simulink model "LV_grid"  (R2021b)
settings: Solver=VariableStepAuto  StartTime=0  StopTime=5.0005  FixedStep=5e-4  RelTol=1e-3
model workspace (MAT data in the model file):
  P2_1 = 3450
  idx = 1
  time_counter = 1
libraries: spsGroundLib x97, spsStairGeneratorLib x96, spsPiSectionLineLib x90, spsThreePhasePISectionLineLib x90, spsVariableInductorLib x48, spsVariableResistorLib x48, spsRMSLib x36, spsThreePhaseVIMeasurementLib x34, spsACVoltageSourceLib x5, spsLinearTransformerLib x5, spsPower3phInstantaneousLib x1, spsThreePhaseMutualInductanceZ1Z0Lib x1
(part 3 of 6)

== system LV_grid/L25 ==
  note: 2.5m
  note: 2.5m
  note: 2.5m
  note: 2.5m
  Ground : spsGroundLib/Ground  LConnTagsString=a
  Ground1 : spsGroundLib/Ground  LConnTagsString=a
  Ground2 : spsGroundLib/Ground  LConnTagsString=a
  L1 : Subsystem
  L2 : Subsystem
  L3 : Subsystem
  L4 : Subsystem
  A : PMIOPort  Side=Left
  B : PMIOPort  Port=2  Side=Left
  C : PMIOPort  Port=3  Side=Left
  N : PMIOPort  Port=4  Side=Left
  a : PMIOPort  Port=5  Side=Right
  b : PMIOPort  Port=6  Side=Right
  c : PMIOPort  Port=7  Side=Right
  n : PMIOPort  Port=8  Side=Right
  connections:
  L1/LConn3 -- C/RConn1
  L3/LConn4 -- Ground1/LConn1 -- L2/RConn4
  L1/LConn4 -- N/RConn1
  L1/LConn2 -- B/RConn1
  L1/LConn1 -- A/RConn1
  L2/LConn4 -- Ground/LConn1 -- L1/RConn4
  L4/LConn4 -- Ground2/LConn1 -- L3/RConn4
  L4/RConn4 -- n/RConn1
  L3/LConn1 -- L2/RConn1
  L3/LConn2 -- L2/RConn2
  L3/LConn3 -- L2/RConn3
  L4/LConn1 -- L3/RConn1
  L4/LConn2 -- L3/RConn2
  L4/LConn3 -- L3/RConn3
  L4/RConn1 -- a/RConn1
  L4/RConn2 -- b/RConn1
  L4/RConn3 -- c/RConn1
  L2/LConn1 -- L1/RConn1
  L2/LConn2 -- L1/RConn2
  L2/LConn3 -- L1/RConn3

== system LV_grid/L26 ==
  note: 2.5m
  note: 2.5m
  Ground : spsGroundLib/Ground  LConnTagsString=a
  L1 : Subsystem
  L2 : Subsystem
  A : PMIOPort  Side=Left
  B : PMIOPort  Port=2  Side=Left
  C : PMIOPort  Port=3  Side=Left
  N : PMIOPort  Port=4  Side=Left
  a : PMIOPort  Port=5  Side=Right
  b : PMIOPort  Port=6  Side=Right
  c : PMIOPort  Port=7  Side=Right
  n : PMIOPort  Port=8  Side=Right
  connections:
  L2/RConn4 -- n/RConn1
  L1/RConn4 -- L2/LConn4 -- Ground/LConn1
  L1/LConn4 -- N/RConn1
  L1/LConn3 -- C/RConn1
  L1/LConn2 -- B/RConn1
  L1/LConn1 -- A/RConn1
  L2/RConn1 -- a/RConn1
  L2/RConn2 -- b/RConn1
  L2/RConn3 -- c/RConn1
  L2/LConn1 -- L1/RConn1
  L2/LConn2 -- L1/RConn2
  L2/LConn3 -- L1/RConn3

== system LV_grid/L27 ==
  note: 2.5m
  note: 2.5m
  Ground : spsGroundLib/Ground  LConnTagsString=a
  L1 : Subsystem
  L2 : Subsystem
  A : PMIOPort  Side=Left
  B : PMIOPort  Port=2  Side=Left
  C : PMIOPort  Port=3  Side=Left
  N : PMIOPort  Port=4  Side=Left
  a : PMIOPort  Port=5  Side=Right
  b : PMIOPort  Port=6  Side=Right
  c : PMIOPort  Port=7  Side=Right
  n : PMIOPort  Port=8  Side=Right
  connections:
  L2/RConn4 -- n/RConn1
  L1/RConn4 -- L2/LConn4 -- Ground/LConn1
  L1/LConn4 -- N/RConn1
  L1/LConn3 -- C/RConn1
  L1/LConn2 -- B/RConn1
  L1/LConn1 -- A/RConn1
  L2/RConn1 -- a/RConn1
  L2/RConn2 -- b/RConn1
  L2/RConn3 -- c/RConn1
  L2/LConn1 -- L1/RConn1
  L2/LConn2 -- L1/RConn2
  L2/LConn3 -- L1/RConn3

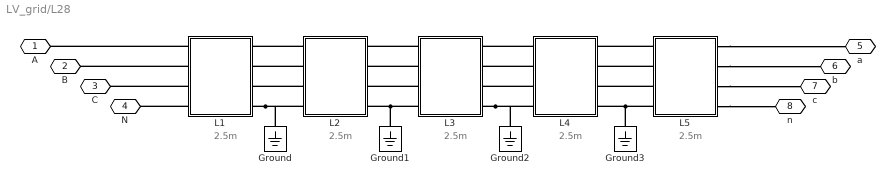
== system LV_grid/L28 ==
  note: 2.5m
  note: 2.5m
  note: 2.5m
  note: 2.5m
  note: 2.5m
  Ground{,1..3} (4 alike) : spsGroundLib/Ground  LConnTagsString=a
  L1 : Subsystem
  L2 : Subsystem
  L3 : Subsystem
  L4 : Subsystem
  L5 : Subsystem
  A : PMIOPort  Side=Left
  B : PMIOPort  Port=2  Side=Left
  C : PMIOPort  Port=3  Side=Left
  N : PMIOPort  Port=4  Side=Left
  a : PMIOPort  Port=5  Side=Right
  b : PMIOPort  Port=6  Side=Right
  c : PMIOPort  Port=7  Side=Right
  n : PMIOPort  Port=8  Side=Right
  connections:
  L1/LConn1 -- A/RConn1
  L1/LConn4 -- N/RConn1
  L1/LConn2 -- B/RConn1
  L1/LConn3 -- C/RConn1
  L5/LConn4 -- L4/RConn4 -- Ground3/LConn1
  L3/RConn4 -- L4/LConn4 -- Ground2/LConn1
  L5/RConn4 -- n/RConn1
  L3/LConn4 -- L2/RConn4 -- Ground1/LConn1
  L1/RConn4 -- L2/LConn4 -- Ground/LConn1
  L3/LConn1 -- L2/RConn1
  L3/LConn2 -- L2/RConn2
  L3/LConn3 -- L2/RConn3
  L5/RConn1 -- a/RConn1
  L5/RConn2 -- b/RConn1
  L5/RConn3 -- c/RConn1
  L5/LConn1 -- L4/RConn1
  L5/LConn2 -- L4/RConn2
  L5/LConn3 -- L4/RConn3
  L4/LConn1 -- L3/RConn1
  L4/LConn2 -- L3/RConn2
  L4/LConn3 -- L3/RConn3
  L2/LConn1 -- L1/RConn1
  L2/LConn2 -- L1/RConn2
  L2/LConn3 -- L1/RConn3

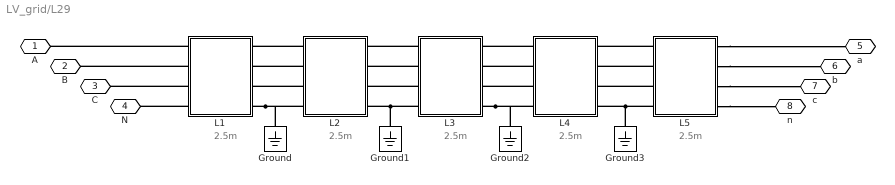
== system LV_grid/L29 ==
  note: 2.5m
  note: 2.5m
  note: 2.5m
  note: 2.5m
  note: 2.5m
  Ground{,1..3} (4 alike) : spsGroundLib/Ground  LConnTagsString=a
  L1 : Subsystem
  L2 : Subsystem
  L3 : Subsystem
  L4 : Subsystem
  L5 : Subsystem
  A : PMIOPort  Side=Left
  B : PMIOPort  Port=2  Side=Left
  C : PMIOPort  Port=3  Side=Left
  N : PMIOPort  Port=4  Side=Left
  a : PMIOPort  Port=5  Side=Right
  b : PMIOPort  Port=6  Side=Right
  c : PMIOPort  Port=7  Side=Right
  n : PMIOPort  Port=8  Side=Right
  connections:
  L1/LConn1 -- A/RConn1
  L1/LConn4 -- N/RConn1
  L1/LConn2 -- B/RConn1
  L1/LConn3 -- C/RConn1
  L5/LConn4 -- L4/RConn4 -- Ground3/LConn1
  L3/RConn4 -- L4/LConn4 -- Ground2/LConn1
  L5/RConn4 -- n/RConn1
  L3/LConn4 -- L2/RConn4 -- Ground1/LConn1
  L1/RConn4 -- L2/LConn4 -- Ground/LConn1
  L4/LConn1 -- L3/RConn1
  L4/LConn2 -- L3/RConn2
  L4/LConn3 -- L3/RConn3
  L5/LConn1 -- L4/RConn1
  L5/LConn2 -- L4/RConn2
  L5/LConn3 -- L4/RConn3
  L2/LConn1 -- L1/RConn1
  L2/LConn2 -- L1/RConn2
  L2/LConn3 -- L1/RConn3
  L5/RConn1 -- a/RConn1
  L5/RConn2 -- b/RConn1
  L5/RConn3 -- c/RConn1
  L3/LConn1 -- L2/RConn1
  L3/LConn2 -- L2/RConn2
  L3/LConn3 -- L2/RConn3

== system LV_grid/L3 ==
  note: 2.5m
  L1 : Subsystem
  A : PMIOPort  Side=Left
  B : PMIOPort  Port=2  Side=Left
  C : PMIOPort  Port=3  Side=Left
  N : PMIOPort  Port=4  Side=Left
  a : PMIOPort  Port=5  Side=Right
  b : PMIOPort  Port=6  Side=Right
  c : PMIOPort  Port=7  Side=Right
  n : PMIOPort  Port=8  Side=Right
  connections:
  B/RConn1 -- L1/LConn2
  n/RConn1 -- L1/RConn4
  C/RConn1 -- L1/LConn3
  N/RConn1 -- L1/LConn4
  A/RConn1 -- L1/LConn1
  L1/RConn1 -- a/RConn1
  L1/RConn2 -- b/RConn1
  L1/RConn3 -- c/RConn1

== system LV_grid/L30 ==
  note: 2.5m
  note: 2.5m
  Ground : spsGroundLib/Ground  LConnTagsString=a
  L1 : Subsystem
  L2 : Subsystem
  A : PMIOPort  Side=Left
  B : PMIOPort  Port=2  Side=Left
  C : PMIOPort  Port=3  Side=Left
  N : PMIOPort  Port=4  Side=Left
  a : PMIOPort  Port=5  Side=Right
  b : PMIOPort  Port=6  Side=Right
  c : PMIOPort  Port=7  Side=Right
  n : PMIOPort  Port=8  Side=Right
  connections:
  L2/RConn4 -- n/RConn1
  L1/RConn4 -- L2/LConn4 -- Ground/LConn1
  L1/LConn4 -- N/RConn1
  L1/LConn3 -- C/RConn1
  L1/LConn2 -- B/RConn1
  L1/LConn1 -- A/RConn1
  L2/LConn1 -- L1/RConn1
  L2/LConn2 -- L1/RConn2
  L2/LConn3 -- L1/RConn3
  L2/RConn1 -- a/RConn1
  L2/RConn2 -- b/RConn1
  L2/RConn3 -- c/RConn1

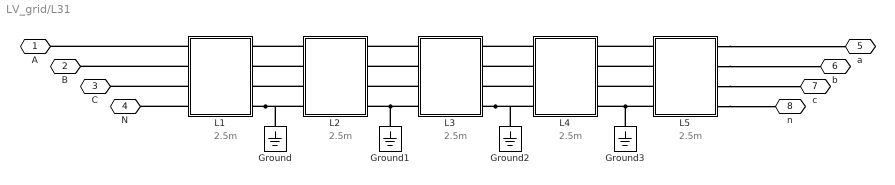
== system LV_grid/L31 ==
  note: 2.5m
  note: 2.5m
  note: 2.5m
  note: 2.5m
  note: 2.5m
  Ground{,1..3} (4 alike) : spsGroundLib/Ground  LConnTagsString=a
  L1 : Subsystem
  L2 : Subsystem
  L3 : Subsystem
  L4 : Subsystem
  L5 : Subsystem
  A : PMIOPort  Side=Left
  B : PMIOPort  Port=2  Side=Left
  C : PMIOPort  Port=3  Side=Left
  N : PMIOPort  Port=4  Side=Left
  a : PMIOPort  Port=5  Side=Right
  b : PMIOPort  Port=6  Side=Right
  c : PMIOPort  Port=7  Side=Right
  n : PMIOPort  Port=8  Side=Right
  connections:
  L1/LConn1 -- A/RConn1
  L1/LConn4 -- N/RConn1
  L1/LConn2 -- B/RConn1
  L1/LConn3 -- C/RConn1
  L5/LConn4 -- L4/RConn4 -- Ground3/LConn1
  L3/RConn4 -- L4/LConn4 -- Ground2/LConn1
  L5/RConn4 -- n/RConn1
  L3/LConn4 -- L2/RConn4 -- Ground1/LConn1
  L1/RConn4 -- L2/LConn4 -- Ground/LConn1
  L5/RConn1 -- a/RConn1
  L5/RConn2 -- b/RConn1
  L5/RConn3 -- c/RConn1
  L3/LConn1 -- L2/RConn1
  L3/LConn2 -- L2/RConn2
  L3/LConn3 -- L2/RConn3
  L2/LConn1 -- L1/RConn1
  L2/LConn2 -- L1/RConn2
  L2/LConn3 -- L1/RConn3
  L5/LConn1 -- L4/RConn1
  L5/LConn2 -- L4/RConn2
  L5/LConn3 -- L4/RConn3
  L4/LConn1 -- L3/RConn1
  L4/LConn2 -- L3/RConn2
  L4/LConn3 -- L3/RConn3

== system LV_grid/L32 ==
  note: 2.5m
  note: 2.5m
  note: 2.5m
  note: 2.5m
  Ground : spsGroundLib/Ground  LConnTagsString=a
  Ground1 : spsGroundLib/Ground  LConnTagsString=a
  Ground2 : spsGroundLib/Ground  LConnTagsString=a
  L1 : Subsystem
  L2 : Subsystem
  L3 : Subsystem
  L4 : Subsystem
  A : PMIOPort  Side=Left
  B : PMIOPort  Port=2  Side=Left
  C : PMIOPort  Port=3  Side=Left
  N : PMIOPort  Port=4  Side=Left
  a : PMIOPort  Port=5  Side=Right
  b : PMIOPort  Port=6  Side=Right
  c : PMIOPort  Port=7  Side=Right
  n : PMIOPort  Port=8  Side=Right
  connections:
  L1/LConn3 -- C/RConn1
  L2/RConn4 -- L3/LConn4 -- Ground1/LConn1
  L1/LConn4 -- N/RConn1
  L1/LConn2 -- B/RConn1
  L1/LConn1 -- A/RConn1
  L1/RConn4 -- L2/LConn4 -- Ground/LConn1
  L3/RConn4 -- L4/LConn4 -- Ground2/LConn1
  L4/RConn4 -- n/RConn1
  L4/RConn1 -- a/RConn1
  L4/RConn2 -- b/RConn1
  L4/RConn3 -- c/RConn1
  L2/LConn1 -- L1/RConn1
  L2/LConn2 -- L1/RConn2
  L2/LConn3 -- L1/RConn3
  L4/LConn1 -- L3/RConn1
  L4/LConn2 -- L3/RConn2
  L4/LConn3 -- L3/RConn3
  L3/LConn1 -- L2/RConn1
  L3/LConn2 -- L2/RConn2
  L3/LConn3 -- L2/RConn3

== system LV_grid/L4 ==
  note: 2.5m
  note: 2.5m
  Ground : spsGroundLib/Ground  LConnTagsString=a
  L1 : Subsystem
  L2 : Subsystem
  A : PMIOPort  Side=Left
  B : PMIOPort  Port=2  Side=Left
  C : PMIOPort  Port=3  Side=Left
  N : PMIOPort  Port=4  Side=Left
  a : PMIOPort  Port=5  Side=Right
  b : PMIOPort  Port=6  Side=Right
  c : PMIOPort  Port=7  Side=Right
  n : PMIOPort  Port=8  Side=Right
  connections:
  L2/RConn4 -- n/RConn1
  L2/LConn4 -- Ground/LConn1 -- L1/RConn4
  L1/LConn4 -- N/RConn1
  L1/LConn3 -- C/RConn1
  L1/LConn2 -- B/RConn1
  L1/LConn1 -- A/RConn1
  L2/LConn1 -- L1/RConn1
  L2/LConn2 -- L1/RConn2
  L2/LConn3 -- L1/RConn3
  L2/RConn1 -- a/RConn1
  L2/RConn2 -- b/RConn1
  L2/RConn3 -- c/RConn1

== system LV_grid/L5 ==
  note: 2.5m
  note: 2.5m
  Ground : spsGroundLib/Ground  LConnTagsString=a
  L1 : Subsystem
  L2 : Subsystem
  A : PMIOPort  Side=Left
  B : PMIOPort  Port=2  Side=Left
  C : PMIOPort  Port=3  Side=Left
  N : PMIOPort  Port=4  Side=Left
  a : PMIOPort  Port=5  Side=Right
  b : PMIOPort  Port=6  Side=Right
  c : PMIOPort  Port=7  Side=Right
  n : PMIOPort  Port=8  Side=Right
  connections:
  L2/RConn4 -- n/RConn1
  L1/RConn4 -- L2/LConn4 -- Ground/LConn1
  L1/LConn4 -- N/RConn1
  L1/LConn3 -- C/RConn1
  L1/LConn2 -- B/RConn1
  L1/LConn1 -- A/RConn1
  L2/LConn1 -- L1/RConn1
  L2/LConn2 -- L1/RConn2
  L2/LConn3 -- L1/RConn3
  L2/RConn1 -- a/RConn1
  L2/RConn2 -- b/RConn1
  L2/RConn3 -- c/RConn1

== system LV_grid/L6 ==
  note: 2.5m
  L1 : Subsystem
  A : PMIOPort  Side=Left
  B : PMIOPort  Port=2  Side=Left
  C : PMIOPort  Port=3  Side=Left
  N : PMIOPort  Port=4  Side=Left
  a : PMIOPort  Port=5  Side=Right
  b : PMIOPort  Port=6  Side=Right
  c : PMIOPort  Port=7  Side=Right
  n : PMIOPort  Port=8  Side=Right
  connections:
  B/RConn1 -- L1/LConn2
  n/RConn1 -- L1/RConn4
  C/RConn1 -- L1/LConn3
  N/RConn1 -- L1/LConn4
  A/RConn1 -- L1/LConn1
  L1/RConn1 -- a/RConn1
  L1/RConn2 -- b/RConn1
  L1/RConn3 -- c/RConn1

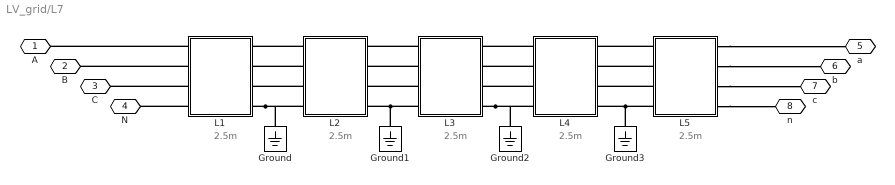
== system LV_grid/L7 ==
  note: 2.5m
  note: 2.5m
  note: 2.5m
  note: 2.5m
  note: 2.5m
  Ground{,1..3} (4 alike) : spsGroundLib/Ground  LConnTagsString=a
  L1 : Subsystem
  L2 : Subsystem
  L3 : Subsystem
  L4 : Subsystem
  L5 : Subsystem
  A : PMIOPort  Side=Left
  B : PMIOPort  Port=2  Side=Left
  C : PMIOPort  Port=3  Side=Left
  N : PMIOPort  Port=4  Side=Left
  a : PMIOPort  Port=5  Side=Right
  b : PMIOPort  Port=6  Side=Right
  c : PMIOPort  Port=7  Side=Right
  n : PMIOPort  Port=8  Side=Right
  connections:
  L1/LConn1 -- A/RConn1
  L1/LConn4 -- N/RConn1
  L1/LConn2 -- B/RConn1
  L1/LConn3 -- C/RConn1
  L5/LConn4 -- L4/RConn4 -- Ground3/LConn1
  L3/RConn4 -- L4/LConn4 -- Ground2/LConn1
  L5/RConn4 -- n/RConn1
  L3/LConn4 -- L2/RConn4 -- Ground1/LConn1
  L1/RConn4 -- L2/LConn4 -- Ground/LConn1
  L3/LConn1 -- L2/RConn1
  L3/LConn2 -- L2/RConn2
  L3/LConn3 -- L2/RConn3
  L5/LConn1 -- L4/RConn1
  L5/LConn2 -- L4/RConn2
  L5/LConn3 -- L4/RConn3
  L5/RConn1 -- a/RConn1
  L5/RConn2 -- b/RConn1
  L5/RConn3 -- c/RConn1
  L4/LConn1 -- L3/RConn1
  L4/LConn2 -- L3/RConn2
  L4/LConn3 -- L3/RConn3
  L2/LConn1 -- L1/RConn1
  L2/LConn2 -- L1/RConn2
  L2/LConn3 -- L1/RConn3

== system LV_grid/L8 ==
  note: 2.5m
  note: 2.5m
  note: 2.5m
  Ground : spsGroundLib/Ground  LConnTagsString=a
  Ground1 : spsGroundLib/Ground  LConnTagsString=a
  L1 : Subsystem
  L2 : Subsystem
  L3 : Subsystem
  A : PMIOPort  Side=Left
  B : PMIOPort  Port=2  Side=Left
  C : PMIOPort  Port=3  Side=Left
  N : PMIOPort  Port=4  Side=Left
  a : PMIOPort  Port=5  Side=Right
  b : PMIOPort  Port=6  Side=Right
  c : PMIOPort  Port=7  Side=Right
  n : PMIOPort  Port=8  Side=Right
  connections:
  L1/LConn2 -- B/RConn1
  L1/LConn4 -- N/RConn1
  L1/LConn1 -- A/RConn1
  L2/LConn4 -- Ground/LConn1 -- L1/RConn4
  L1/LConn3 -- C/RConn1
  L3/RConn4 -- n/RConn1
  L3/LConn4 -- Ground1/LConn1 -- L2/RConn4
  L3/RConn1 -- a/RConn1
  L3/RConn2 -- b/RConn1
  L3/RConn3 -- c/RConn1
  L3/LConn1 -- L2/RConn1
  L3/LConn2 -- L2/RConn2
  L3/LConn3 -- L2/RConn3
  L2/LConn1 -- L1/RConn1
  L2/LConn2 -- L1/RConn2
  L2/LConn3 -- L1/RConn3

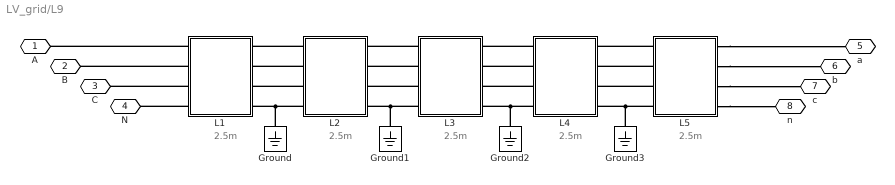
== system LV_grid/L9 ==
  note: 2.5m
  note: 2.5m
  note: 2.5m
  note: 2.5m
  note: 2.5m
  Ground{,1..3} (4 alike) : spsGroundLib/Ground  LConnTagsString=a
  L1 : Subsystem
  L2 : Subsystem
  L3 : Subsystem
  L4 : Subsystem
  L5 : Subsystem
  A : PMIOPort  Side=Left
  B : PMIOPort  Port=2  Side=Left
  C : PMIOPort  Port=3  Side=Left
  N : PMIOPort  Port=4  Side=Left
  a : PMIOPort  Port=5  Side=Right
  b : PMIOPort  Port=6  Side=Right
  c : PMIOPort  Port=7  Side=Right
  n : PMIOPort  Port=8  Side=Right
  connections:
  L1/LConn1 -- A/RConn1
  L1/LConn4 -- N/RConn1
  L1/LConn2 -- B/RConn1
  L1/LConn3 -- C/RConn1
  L5/LConn4 -- Ground3/LConn1 -- L4/RConn4
  L4/LConn4 -- Ground2/LConn1 -- L3/RConn4
  L5/RConn4 -- n/RConn1
  L3/LConn4 -- Ground1/LConn1 -- L2/RConn4
  L2/LConn4 -- Ground/LConn1 -- L1/RConn4
  L5/LConn1 -- L4/RConn1
  L5/LConn2 -- L4/RConn2
  L5/LConn3 -- L4/RConn3
  L5/RConn1 -- a/RConn1
  L5/RConn2 -- b/RConn1
  L5/RConn3 -- c/RConn1
  L4/LConn1 -- L3/RConn1
  L4/LConn2 -- L3/RConn2
  L4/LConn3 -- L3/RConn3
  L2/LConn1 -- L1/RConn1
  L2/LConn2 -- L1/RConn2
  L2/LConn3 -- L1/RConn3
  L3/LConn1 -- L2/RConn1
  L3/LConn2 -- L2/RConn2
  L3/LConn3 -- L2/RConn3

== system LV_grid/RL_Load ==
  L_signal : Inport
  R_signal : Inport  Port=2
  Variable Inductor : spsVariableInductorLib/Variable Inductor  methode=Backward Euler  Labsmin=0.06  Initialize=off  iL0=0  L0=1e-3  Vl0=-0.057039
      settings: SourceProductBaseCode=PS
  Variable Resistor : spsVariableResistorLib/Variable Resistor  Rabsmin=20
      settings: SourceProductBaseCode=PS
  V+ : PMIOPort  Side=Right
  V- : PMIOPort  Port=2  Side=Right
  wires:
  R_signal/1 -> Variable Resistor/1
  L_signal/1 -> Variable Inductor/1
  connections:
  Variable Inductor/LConn1 -- Variable Resistor/LConn1 -- V+/RConn1
  Variable Resistor/RConn1 -- Variable Inductor/RConn1 -- V-/RConn1

== system LV_grid/RL_Load1 ==
  L_signal : Inport
  R_signal : Inport  Port=2
  Variable Inductor : spsVariableInductorLib/Variable Inductor  methode=Backward Euler  Labsmin=0.06  Initialize=off  iL0=0  L0=1e-3  Vl0=-282.7103
      settings: SourceProductBaseCode=PS
  Variable Resistor : spsVariableResistorLib/Variable Resistor  Rabsmin=20
      settings: SourceProductBaseCode=PS
  V+ : PMIOPort  Side=Right
  V- : PMIOPort  Port=2  Side=Right
  wires:
  R_signal/1 -> Variable Resistor/1
  L_signal/1 -> Variable Inductor/1
  connections:
  Variable Inductor/LConn1 -- V+/RConn1 -- Variable Resistor/LConn1
  V-/RConn1 -- Variable Resistor/RConn1 -- Variable Inductor/RConn1

== system LV_grid/RL_Load10 ==
  L_signal : Inport
  R_signal : Inport  Port=2
  Variable Inductor : spsVariableInductorLib/Variable Inductor  methode=Backward Euler  Labsmin=0.06  Initialize=off  iL0=0  L0=1e-3  Vl0=-0.056313
      settings: SourceProductBaseCode=PS
  Variable Resistor : spsVariableResistorLib/Variable Resistor  Rabsmin=20
      settings: SourceProductBaseCode=PS
  V+ : PMIOPort  Side=Right
  V- : PMIOPort  Port=2  Side=Right
  wires:
  R_signal/1 -> Variable Resistor/1
  L_signal/1 -> Variable Inductor/1
  connections:
  Variable Inductor/LConn1 -- V+/RConn1 -- Variable Resistor/LConn1
  V-/RConn1 -- Variable Resistor/RConn1 -- Variable Inductor/RConn1

== system LV_grid/RL_Load11 ==
  L_signal : Inport
  R_signal : Inport  Port=2
  Variable Inductor : spsVariableInductorLib/Variable Inductor  methode=Backward Euler  Labsmin=0.06  Initialize=off  iL0=0  L0=1e-3  Vl0=-282.6497
      settings: SourceProductBaseCode=PS
  Variable Resistor : spsVariableResistorLib/Variable Resistor  Rabsmin=20
      settings: SourceProductBaseCode=PS
  V+ : PMIOPort  Side=Right
  V- : PMIOPort  Port=2  Side=Right
  wires:
  R_signal/1 -> Variable Resistor/1
  L_signal/1 -> Variable Inductor/1
  connections:
  Variable Inductor/LConn1 -- V+/RConn1 -- Variable Resistor/LConn1
  V-/RConn1 -- Variable Resistor/RConn1 -- Variable Inductor/RConn1

== system LV_grid/RL_Load12 ==
  L_signal : Inport
  R_signal : Inport  Port=2
  Variable Inductor : spsVariableInductorLib/Variable Inductor  methode=Backward Euler  Labsmin=0.06  Initialize=off  iL0=0  L0=1e-3  Vl0=-0.057253
      settings: SourceProductBaseCode=PS
  Variable Resistor : spsVariableResistorLib/Variable Resistor  Rabsmin=20
      settings: SourceProductBaseCode=PS
  V+ : PMIOPort  Side=Right
  V- : PMIOPort  Port=2  Side=Right
  wires:
  R_signal/1 -> Variable Resistor/1
  L_signal/1 -> Variable Inductor/1
  connections:
  Variable Inductor/LConn1 -- V+/RConn1 -- Variable Resistor/LConn1
  V-/RConn1 -- Variable Resistor/RConn1 -- Variable Inductor/RConn1

== system LV_grid/RL_Load13 ==
  L_signal : Inport
  R_signal : Inport  Port=2
  Variable Inductor : spsVariableInductorLib/Variable Inductor  methode=Backward Euler  Labsmin=0.06  Initialize=off  iL0=0  L0=1e-3  Vl0=282.7771
      settings: SourceProductBaseCode=PS
  Variable Resistor : spsVariableResistorLib/Variable Resistor  Rabsmin=20
      settings: SourceProductBaseCode=PS
  V+ : PMIOPort  Side=Right
  V- : PMIOPort  Port=2  Side=Right
  wires:
  R_signal/1 -> Variable Resistor/1
  L_signal/1 -> Variable Inductor/1
  connections:
  Variable Inductor/LConn1 -- V+/RConn1 -- Variable Resistor/LConn1
  V-/RConn1 -- Variable Resistor/RConn1 -- Variable Inductor/RConn1

== system LV_grid/RL_Load14 ==
  L_signal : Inport
  R_signal : Inport  Port=2
  Variable Inductor : spsVariableInductorLib/Variable Inductor  methode=Backward Euler  Labsmin=0.06  Initialize=off  iL0=0  L0=1e-3  Vl0=-282.6947
      settings: SourceProductBaseCode=PS
  Variable Resistor : spsVariableResistorLib/Variable Resistor  Rabsmin=20
      settings: SourceProductBaseCode=PS
  V+ : PMIOPort  Side=Right
  V- : PMIOPort  Port=2  Side=Right
  wires:
  R_signal/1 -> Variable Resistor/1
  L_signal/1 -> Variable Inductor/1
  connections:
  Variable Inductor/LConn1 -- V+/RConn1 -- Variable Resistor/LConn1
  V-/RConn1 -- Variable Resistor/RConn1 -- Variable Inductor/RConn1

== system LV_grid/RL_Load15 ==
  L_signal : Inport
  R_signal : Inport  Port=2
  Variable Inductor : spsVariableInductorLib/Variable Inductor  methode=Backward Euler  Labsmin=0.06  Initialize=off  iL0=0  L0=1e-3  Vl0=-0.057253
      settings: SourceProductBaseCode=PS
  Variable Resistor : spsVariableResistorLib/Variable Resistor  Rabsmin=20
      settings: SourceProductBaseCode=PS
  V+ : PMIOPort  Side=Right
  V- : PMIOPort  Port=2  Side=Right
  wires:
  R_signal/1 -> Variable Resistor/1
  L_signal/1 -> Variable Inductor/1
  connections:
  Variable Inductor/LConn1 -- V+/RConn1 -- Variable Resistor/LConn1
  V-/RConn1 -- Variable Resistor/RConn1 -- Variable Inductor/RConn1

== system LV_grid/RL_Load16 ==
  L_signal : Inport
  R_signal : Inport  Port=2
  Variable Inductor : spsVariableInductorLib/Variable Inductor  methode=Backward Euler  Labsmin=0.06  Initialize=off  iL0=0  L0=1e-3  Vl0=-282.6933
      settings: SourceProductBaseCode=PS
  Variable Resistor : spsVariableResistorLib/Variable Resistor  Rabsmin=20
      settings: SourceProductBaseCode=PS
  V+ : PMIOPort  Side=Right
  V- : PMIOPort  Port=2  Side=Right
  wires:
  R_signal/1 -> Variable Resistor/1
  L_signal/1 -> Variable Inductor/1
  connections:
  Variable Inductor/LConn1 -- V+/RConn1 -- Variable Resistor/LConn1
  V-/RConn1 -- Variable Resistor/RConn1 -- Variable Inductor/RConn1

== system LV_grid/RL_Load17 ==
  L_signal : Inport
  R_signal : Inport  Port=2
  Variable Inductor : spsVariableInductorLib/Variable Inductor  methode=Backward Euler  Labsmin=0.06  Initialize=off  iL0=0  L0=1e-3  Vl0=282.7771
      settings: SourceProductBaseCode=PS
  Variable Resistor : spsVariableResistorLib/Variable Resistor  Rabsmin=20
      settings: SourceProductBaseCode=PS
  V+ : PMIOPort  Side=Right
  V- : PMIOPort  Port=2  Side=Right
  wires:
  R_signal/1 -> Variable Resistor/1
  L_signal/1 -> Variable Inductor/1
  connections:
  Variable Inductor/LConn1 -- V+/RConn1 -- Variable Resistor/LConn1
  V-/RConn1 -- Variable Resistor/RConn1 -- Variable Inductor/RConn1

== system LV_grid/RL_Load18 ==
  L_signal : Inport
  R_signal : Inport  Port=2
  Variable Inductor : spsVariableInductorLib/Variable Inductor  methode=Backward Euler  Labsmin=0.06  Initialize=off  iL0=0  L0=1e-3  Vl0=-282.7103
      settings: SourceProductBaseCode=PS
  Variable Resistor : spsVariableResistorLib/Variable Resistor  Rabsmin=20
      settings: SourceProductBaseCode=PS
  V+ : PMIOPort  Side=Right
  V- : PMIOPort  Port=2  Side=Right
  wires:
  R_signal/1 -> Variable Resistor/1
  L_signal/1 -> Variable Inductor/1
  connections:
  Variable Inductor/LConn1 -- V+/RConn1 -- Variable Resistor/LConn1
  V-/RConn1 -- Variable Resistor/RConn1 -- Variable Inductor/RConn1

== system LV_grid/RL_Load19 ==
  L_signal : Inport
  R_signal : Inport  Port=2
  Variable Inductor : spsVariableInductorLib/Variable Inductor  methode=Backward Euler  Labsmin=0.06  Initialize=off  iL0=0  L0=1e-3  Vl0=-0.05675
      settings: SourceProductBaseCode=PS
  Variable Resistor : spsVariableResistorLib/Variable Resistor  Rabsmin=20
      settings: SourceProductBaseCode=PS
  V+ : PMIOPort  Side=Right
  V- : PMIOPort  Port=2  Side=Right
  wires:
  R_signal/1 -> Variable Resistor/1
  L_signal/1 -> Variable Inductor/1
  connections:
  Variable Inductor/LConn1 -- V+/RConn1 -- Variable Resistor/LConn1
  V-/RConn1 -- Variable Resistor/RConn1 -- Variable Inductor/RConn1

== system LV_grid/RL_Load2 ==
  L_signal : Inport
  R_signal : Inport  Port=2
  Variable Inductor : spsVariableInductorLib/Variable Inductor  methode=Backward Euler  Labsmin=0.06  Initialize=off  iL0=0  L0=1e-3  Vl0=282.7771
      settings: SourceProductBaseCode=PS
  Variable Resistor : spsVariableResistorLib/Variable Resistor  Rabsmin=20
      settings: SourceProductBaseCode=PS
  V+ : PMIOPort  Side=Right
  V- : PMIOPort  Port=2  Side=Right
  wires:
  R_signal/1 -> Variable Resistor/1
  L_signal/1 -> Variable Inductor/1
  connections:
  Variable Inductor/LConn1 -- V+/RConn1 -- Variable Resistor/LConn1
  V-/RConn1 -- Variable Resistor/RConn1 -- Variable Inductor/RConn1

== system LV_grid/RL_Load20 ==
  L_signal : Inport
  R_signal : Inport  Port=2
  Variable Inductor : spsVariableInductorLib/Variable Inductor  methode=Backward Euler  Labsmin=0.06  Initialize=off  iL0=0  L0=1e-3  Vl0=-282.6598
      settings: SourceProductBaseCode=PS
  Variable Resistor : spsVariableResistorLib/Variable Resistor  Rabsmin=20
      settings: SourceProductBaseCode=PS
  V+ : PMIOPort  Side=Right
  V- : PMIOPort  Port=2  Side=Right
  wires:
  R_signal/1 -> Variable Resistor/1
  L_signal/1 -> Variable Inductor/1
  connections:
  Variable Inductor/LConn1 -- V+/RConn1 -- Variable Resistor/LConn1
  V-/RConn1 -- Variable Resistor/RConn1 -- Variable Inductor/RConn1

== system LV_grid/RL_Load21 ==
  L_signal : Inport
  R_signal : Inport  Port=2
  Variable Inductor : spsVariableInductorLib/Variable Inductor  methode=Backward Euler  Labsmin=0.06  Initialize=off  iL0=0  L0=1e-3  Vl0=282.8043
      settings: SourceProductBaseCode=PS
  Variable Resistor : spsVariableResistorLib/Variable Resistor  Rabsmin=20
      settings: SourceProductBaseCode=PS
  V+ : PMIOPort  Side=Right
  V- : PMIOPort  Port=2  Side=Right
  wires:
  R_signal/1 -> Variable Resistor/1
  L_signal/1 -> Variable Inductor/1
  connections:
  Variable Inductor/LConn1 -- V+/RConn1 -- Variable Resistor/LConn1
  V-/RConn1 -- Variable Resistor/RConn1 -- Variable Inductor/RConn1

== system LV_grid/RL_Load22 ==
  L_signal : Inport
  R_signal : Inport  Port=2
  Variable Inductor : spsVariableInductorLib/Variable Inductor  methode=Backward Euler  Labsmin=0.06  Initialize=off  iL0=0  L0=1e-3  Vl0=-282.6348
      settings: SourceProductBaseCode=PS
  Variable Resistor : spsVariableResistorLib/Variable Resistor  Rabsmin=20
      settings: SourceProductBaseCode=PS
  V+ : PMIOPort  Side=Right
  V- : PMIOPort  Port=2  Side=Right
  wires:
  R_signal/1 -> Variable Resistor/1
  L_signal/1 -> Variable Inductor/1
  connections:
  Variable Inductor/LConn1 -- V+/RConn1 -- Variable Resistor/LConn1
  V-/RConn1 -- Variable Resistor/RConn1 -- Variable Inductor/RConn1

== system LV_grid/RL_Load23 ==
  L_signal : Inport
  R_signal : Inport  Port=2
  Variable Inductor : spsVariableInductorLib/Variable Inductor  methode=Backward Euler  Labsmin=0.06  Initialize=off  iL0=0  L0=1e-3  Vl0=-0.056745
      settings: SourceProductBaseCode=PS
  Variable Resistor : spsVariableResistorLib/Variable Resistor  Rabsmin=20
      settings: SourceProductBaseCode=PS
  V+ : PMIOPort  Side=Right
  V- : PMIOPort  Port=2  Side=Right
  wires:
  R_signal/1 -> Variable Resistor/1
  L_signal/1 -> Variable Inductor/1
  connections:
  Variable Inductor/LConn1 -- V+/RConn1 -- Variable Resistor/LConn1
  V-/RConn1 -- Variable Resistor/RConn1 -- Variable Inductor/RConn1

== system LV_grid/RL_Load24 ==
  L_signal : Inport
  R_signal : Inport  Port=2
  Variable Inductor : spsVariableInductorLib/Variable Inductor  methode=Backward Euler  Labsmin=0.06  Initialize=off  iL0=0  L0=1e-3  Vl0=282.8029
      settings: SourceProductBaseCode=PS
  Variable Resistor : spsVariableResistorLib/Variable Resistor  Rabsmin=20
      settings: SourceProductBaseCode=PS
  V+ : PMIOPort  Side=Right
  V- : PMIOPort  Port=2  Side=Right
  wires:
  R_signal/1 -> Variable Resistor/1
  L_signal/1 -> Variable Inductor/1
  connections:
  Variable Inductor/LConn1 -- V+/RConn1 -- Variable Resistor/LConn1
  V-/RConn1 -- Variable Resistor/RConn1 -- Variable Inductor/RConn1

== system LV_grid/RL_Load25 ==
  L_signal : Inport
  R_signal : Inport  Port=2
  Variable Inductor : spsVariableInductorLib/Variable Inductor  methode=Backward Euler  Labsmin=0.06  Initialize=off  iL0=0  L0=1e-3  Vl0=-282.696
      settings: SourceProductBaseCode=PS
  Variable Resistor : spsVariableResistorLib/Variable Resistor  Rabsmin=20
      settings: SourceProductBaseCode=PS
  V+ : PMIOPort  Side=Right
  V- : PMIOPort  Port=2  Side=Right
  wires:
  R_signal/1 -> Variable Resistor/1
  L_signal/1 -> Variable Inductor/1
  connections:
  Variable Inductor/LConn1 -- V+/RConn1 -- Variable Resistor/LConn1
  V-/RConn1 -- Variable Resistor/RConn1 -- Variable Inductor/RConn1

== system LV_grid/RL_Load26 ==
  L_signal : Inport
  R_signal : Inport  Port=2
  Variable Inductor : spsVariableInductorLib/Variable Inductor  methode=Backward Euler  Labsmin=0.06  Initialize=off  iL0=0  L0=1e-3  Vl0=282.6909
      settings: SourceProductBaseCode=PS
  Variable Resistor : spsVariableResistorLib/Variable Resistor  Rabsmin=20
      settings: SourceProductBaseCode=PS
  V+ : PMIOPort  Side=Right
  V- : PMIOPort  Port=2  Side=Right
  wires:
  R_signal/1 -> Variable Resistor/1
  L_signal/1 -> Variable Inductor/1
  connections:
  Variable Inductor/LConn1 -- V+/RConn1 -- Variable Resistor/LConn1
  V-/RConn1 -- Variable Resistor/RConn1 -- Variable Inductor/RConn1

== system LV_grid/RL_Load27 ==
  L_signal : Inport
  R_signal : Inport  Port=2
  Variable Inductor : spsVariableInductorLib/Variable Inductor  methode=Backward Euler  Labsmin=0.06  Initialize=off  iL0=0  L0=1e-3  Vl0=-282.6933
      settings: SourceProductBaseCode=PS
  Variable Resistor : spsVariableResistorLib/Variable Resistor  Rabsmin=20
      settings: SourceProductBaseCode=PS
  V+ : PMIOPort  Side=Right
  V- : PMIOPort  Port=2  Side=Right
  wires:
  R_signal/1 -> Variable Resistor/1
  L_signal/1 -> Variable Inductor/1
  connections:
  Variable Inductor/LConn1 -- V+/RConn1 -- Variable Resistor/LConn1
  V-/RConn1 -- Variable Resistor/RConn1 -- Variable Inductor/RConn1

== system LV_grid/RL_Load28 ==
  L_signal : Inport
  R_signal : Inport  Port=2
  Variable Inductor : spsVariableInductorLib/Variable Inductor  methode=Backward Euler  Labsmin=0.06  Initialize=off  iL0=0  L0=1e-3  Vl0=282.7771
      settings: SourceProductBaseCode=PS
  Variable Resistor : spsVariableResistorLib/Variable Resistor  Rabsmin=20
      settings: SourceProductBaseCode=PS
  V+ : PMIOPort  Side=Right
  V- : PMIOPort  Port=2  Side=Right
  wires:
  R_signal/1 -> Variable Resistor/1
  L_signal/1 -> Variable Inductor/1
  connections:
  Variable Inductor/LConn1 -- V+/RConn1 -- Variable Resistor/LConn1
  V-/RConn1 -- Variable Resistor/RConn1 -- Variable Inductor/RConn1

== system LV_grid/RL_Load29 ==
  L_signal : Inport
  R_signal : Inport  Port=2
  Variable Inductor : spsVariableInductorLib/Variable Inductor  methode=Backward Euler  Labsmin=0.06  Initialize=off  iL0=0  L0=1e-3  Vl0=-282.7103
      settings: SourceProductBaseCode=PS
  Variable Resistor : spsVariableResistorLib/Variable Resistor  Rabsmin=20
      settings: SourceProductBaseCode=PS
  V+ : PMIOPort  Side=Right
  V- : PMIOPort  Port=2  Side=Right
  wires:
  R_signal/1 -> Variable Resistor/1
  L_signal/1 -> Variable Inductor/1
  connections:
  Variable Inductor/LConn1 -- V+/RConn1 -- Variable Resistor/LConn1
  V-/RConn1 -- Variable Resistor/RConn1 -- Variable Inductor/RConn1

== system LV_grid/RL_Load3 ==
  L_signal : Inport
  R_signal : Inport  Port=2
  Variable Inductor : spsVariableInductorLib/Variable Inductor  methode=Backward Euler  Labsmin=0.06  Initialize=off  iL0=0  L0=1e-3  Vl0=-0.05675
      settings: SourceProductBaseCode=PS
  Variable Resistor : spsVariableResistorLib/Variable Resistor  Rabsmin=20
      settings: SourceProductBaseCode=PS
  V+ : PMIOPort  Side=Right
  V- : PMIOPort  Port=2  Side=Right
  wires:
  R_signal/1 -> Variable Resistor/1
  L_signal/1 -> Variable Inductor/1
  connections:
  Variable Inductor/LConn1 -- V+/RConn1 -- Variable Resistor/LConn1
  V-/RConn1 -- Variable Resistor/RConn1 -- Variable Inductor/RConn1

== system LV_grid/RL_Load30 ==
  L_signal : Inport
  R_signal : Inport  Port=2
  Variable Inductor : spsVariableInductorLib/Variable Inductor  methode=Backward Euler  Labsmin=0.06  Initialize=off  iL0=0  L0=1e-3  Vl0=-282.7176
      settings: SourceProductBaseCode=PS
  Variable Resistor : spsVariableResistorLib/Variable Resistor  Rabsmin=20
      settings: SourceProductBaseCode=PS
  V+ : PMIOPort  Side=Right
  V- : PMIOPort  Port=2  Side=Right
  wires:
  R_signal/1 -> Variable Resistor/1
  L_signal/1 -> Variable Inductor/1
  connections:
  Variable Inductor/LConn1 -- V+/RConn1 -- Variable Resistor/LConn1
  V-/RConn1 -- Variable Resistor/RConn1 -- Variable Inductor/RConn1

== system LV_grid/RL_Load31 ==
  L_signal : Inport
  R_signal : Inport  Port=2
  Variable Inductor : spsVariableInductorLib/Variable Inductor  methode=Backward Euler  Labsmin=0.06  Initialize=off  iL0=0  L0=1e-3  Vl0=-282.7182
      settings: SourceProductBaseCode=PS
  Variable Resistor : spsVariableResistorLib/Variable Resistor  Rabsmin=20
      settings: SourceProductBaseCode=PS
  V+ : PMIOPort  Side=Right
  V- : PMIOPort  Port=2  Side=Right
  wires:
  R_signal/1 -> Variable Resistor/1
  L_signal/1 -> Variable Inductor/1
  connections:
  Variable Inductor/LConn1 -- V+/RConn1 -- Variable Resistor/LConn1
  V-/RConn1 -- Variable Resistor/RConn1 -- Variable Inductor/RConn1

== system LV_grid/RL_Load32 ==
  L_signal : Inport
  R_signal : Inport  Port=2
  Variable Inductor : spsVariableInductorLib/Variable Inductor  methode=Backward Euler  Labsmin=0.06  Initialize=off  iL0=0  L0=1e-3  Vl0=282.8035
      settings: SourceProductBaseCode=PS
  Variable Resistor : spsVariableResistorLib/Variable Resistor  Rabsmin=20
      settings: SourceProductBaseCode=PS
  V+ : PMIOPort  Side=Right
  V- : PMIOPort  Port=2  Side=Right
  wires:
  R_signal/1 -> Variable Resistor/1
  L_signal/1 -> Variable Inductor/1
  connections:
  Variable Inductor/LConn1 -- V+/RConn1 -- Variable Resistor/LConn1
  V-/RConn1 -- Variable Resistor/RConn1 -- Variable Inductor/RConn1

== system LV_grid/RL_Load33 ==
  L_signal : Inport
  R_signal : Inport  Port=2
  Variable Inductor : spsVariableInductorLib/Variable Inductor  methode=Backward Euler  Labsmin=0.06  Initialize=off  iL0=0  L0=1e-3  Vl0=282.8026
      settings: SourceProductBaseCode=PS
  Variable Resistor : spsVariableResistorLib/Variable Resistor  Rabsmin=20
      settings: SourceProductBaseCode=PS
  V+ : PMIOPort  Side=Right
  V- : PMIOPort  Port=2  Side=Right
  wires:
  R_signal/1 -> Variable Resistor/1
  L_signal/1 -> Variable Inductor/1
  connections:
  Variable Inductor/LConn1 -- V+/RConn1 -- Variable Resistor/LConn1
  V-/RConn1 -- Variable Resistor/RConn1 -- Variable Inductor/RConn1

== system LV_grid/RL_Load34 ==
  L_signal : Inport
  R_signal : Inport  Port=2
  Variable Inductor : spsVariableInductorLib/Variable Inductor  methode=Backward Euler  Labsmin=0.06  Initialize=off  iL0=0  L0=1e-3  Vl0=-282.6015
      settings: SourceProductBaseCode=PS
  Variable Resistor : spsVariableResistorLib/Variable Resistor  Rabsmin=20
      settings: SourceProductBaseCode=PS
  V+ : PMIOPort  Side=Right
  V- : PMIOPort  Port=2  Side=Right
  wires:
  R_signal/1 -> Variable Resistor/1
  L_signal/1 -> Variable Inductor/1
  connections:
  Variable Inductor/LConn1 -- V+/RConn1 -- Variable Resistor/LConn1
  V-/RConn1 -- Variable Resistor/RConn1 -- Variable Inductor/RConn1

== system LV_grid/RL_Load35 ==
  L_signal : Inport
  R_signal : Inport  Port=2
  Variable Inductor : spsVariableInductorLib/Variable Inductor  methode=Backward Euler  Labsmin=0.06  Initialize=off  iL0=0  L0=1e-3  Vl0=-282.7182
      settings: SourceProductBaseCode=PS
  Variable Resistor : spsVariableResistorLib/Variable Resistor  Rabsmin=20
      settings: SourceProductBaseCode=PS
  V+ : PMIOPort  Side=Right
  V- : PMIOPort  Port=2  Side=Right
  wires:
  R_signal/1 -> Variable Resistor/1
  L_signal/1 -> Variable Inductor/1
  connections:
  Variable Inductor/LConn1 -- V+/RConn1 -- Variable Resistor/LConn1
  V-/RConn1 -- Variable Resistor/RConn1 -- Variable Inductor/RConn1

== system LV_grid/RL_Load36 ==
  L_signal : Inport
  R_signal : Inport  Port=2
  Variable Inductor : spsVariableInductorLib/Variable Inductor  methode=Backward Euler  Labsmin=0.06  Initialize=off  iL0=0  L0=1e-3  Vl0=282.8029
      settings: SourceProductBaseCode=PS
  Variable Resistor : spsVariableResistorLib/Variable Resistor  Rabsmin=20
      settings: SourceProductBaseCode=PS
  V+ : PMIOPort  Side=Right
  V- : PMIOPort  Port=2  Side=Right
  wires:
  R_signal/1 -> Variable Resistor/1
  L_signal/1 -> Variable Inductor/1
  connections:
  Variable Inductor/LConn1 -- V+/RConn1 -- Variable Resistor/LConn1
  V-/RConn1 -- Variable Resistor/RConn1 -- Variable Inductor/RConn1

== system LV_grid/RL_Load37 ==
  L_signal : Inport
  R_signal : Inport  Port=2
  Variable Inductor : spsVariableInductorLib/Variable Inductor  methode=Backward Euler  Labsmin=0.06  Initialize=off  iL0=0  L0=1e-3  Vl0=282.8055
      settings: SourceProductBaseCode=PS
  Variable Resistor : spsVariableResistorLib/Variable Resistor  Rabsmin=20
      settings: SourceProductBaseCode=PS
  V+ : PMIOPort  Side=Right
  V- : PMIOPort  Port=2  Side=Right
  wires:
  R_signal/1 -> Variable Resistor/1
  L_signal/1 -> Variable Inductor/1
  connections:
  Variable Inductor/LConn1 -- V+/RConn1 -- Variable Resistor/LConn1
  V-/RConn1 -- Variable Resistor/RConn1 -- Variable Inductor/RConn1

== system LV_grid/RL_Load38 ==
  L_signal : Inport
  R_signal : Inport  Port=2
  Variable Inductor : spsVariableInductorLib/Variable Inductor  methode=Backward Euler  Labsmin=0.06  Initialize=off  iL0=0  L0=1e-3  Vl0=-0.058139
      settings: SourceProductBaseCode=PS
  Variable Resistor : spsVariableResistorLib/Variable Resistor  Rabsmin=20
      settings: SourceProductBaseCode=PS
  V+ : PMIOPort  Side=Right
  V- : PMIOPort  Port=2  Side=Right
  wires:
  R_signal/1 -> Variable Resistor/1
  L_signal/1 -> Variable Inductor/1
  connections:
  Variable Inductor/LConn1 -- V+/RConn1 -- Variable Resistor/LConn1
  V-/RConn1 -- Variable Resistor/RConn1 -- Variable Inductor/RConn1

== system LV_grid/RL_Load39 ==
  L_signal : Inport
  R_signal : Inport  Port=2
  Variable Inductor : spsVariableInductorLib/Variable Inductor  methode=Backward Euler  Labsmin=0.06  Initialize=off  iL0=0  L0=1e-3  Vl0=-282.6941
      settings: SourceProductBaseCode=PS
  Variable Resistor : spsVariableResistorLib/Variable Resistor  Rabsmin=20
      settings: SourceProductBaseCode=PS
  V+ : PMIOPort  Side=Right
  V- : PMIOPort  Port=2  Side=Right
  wires:
  R_signal/1 -> Variable Resistor/1
  L_signal/1 -> Variable Inductor/1
  connections:
  Variable Inductor/LConn1 -- V+/RConn1 -- Variable Resistor/LConn1
  V-/RConn1 -- Variable Resistor/RConn1 -- Variable Inductor/RConn1

== system LV_grid/RL_Load4 ==
  L_signal : Inport
  R_signal : Inport  Port=2
  Variable Inductor : spsVariableInductorLib/Variable Inductor  methode=Backward Euler  Labsmin=0.06  Initialize=off  iL0=0  L0=1e-3  Vl0=-0.056567
      settings: SourceProductBaseCode=PS
  Variable Resistor : spsVariableResistorLib/Variable Resistor  Rabsmin=20
      settings: SourceProductBaseCode=PS
  V+ : PMIOPort  Side=Right
  V- : PMIOPort  Port=2  Side=Right
  wires:
  R_signal/1 -> Variable Resistor/1
  L_signal/1 -> Variable Inductor/1
  connections:
  Variable Inductor/LConn1 -- V+/RConn1 -- Variable Resistor/LConn1
  V-/RConn1 -- Variable Resistor/RConn1 -- Variable Inductor/RConn1

== system LV_grid/RL_Load40 ==
  L_signal : Inport
  R_signal : Inport  Port=2
  Variable Inductor : spsVariableInductorLib/Variable Inductor  methode=Backward Euler  Labsmin=0.06  Initialize=off  iL0=0  L0=1e-3  Vl0=282.7512
      settings: SourceProductBaseCode=PS
  Variable Resistor : spsVariableResistorLib/Variable Resistor  Rabsmin=20
      settings: SourceProductBaseCode=PS
  V+ : PMIOPort  Side=Right
  V- : PMIOPort  Port=2  Side=Right
  wires:
  R_signal/1 -> Variable Resistor/1
  L_signal/1 -> Variable Inductor/1
  connections:
  Variable Inductor/LConn1 -- V+/RConn1 -- Variable Resistor/LConn1
  V-/RConn1 -- Variable Resistor/RConn1 -- Variable Inductor/RConn1

== system LV_grid/RL_Load41 ==
  L_signal : Inport
  R_signal : Inport  Port=2
  Variable Inductor : spsVariableInductorLib/Variable Inductor  methode=Backward Euler  Labsmin=0.06  Initialize=off  iL0=0  L0=1e-3  Vl0=-0.060204
      settings: SourceProductBaseCode=PS
  Variable Resistor : spsVariableResistorLib/Variable Resistor  Rabsmin=20
      settings: SourceProductBaseCode=PS
  V+ : PMIOPort  Side=Right
  V- : PMIOPort  Port=2  Side=Right
  wires:
  R_signal/1 -> Variable Resistor/1
  L_signal/1 -> Variable Inductor/1
  connections:
  Variable Inductor/LConn1 -- V+/RConn1 -- Variable Resistor/LConn1
  V-/RConn1 -- Variable Resistor/RConn1 -- Variable Inductor/RConn1

== system LV_grid/RL_Load42 ==
  L_signal : Inport
  R_signal : Inport  Port=2
  Variable Inductor : spsVariableInductorLib/Variable Inductor  methode=Backward Euler  Labsmin=0.06  Initialize=off  iL0=0  L0=1e-3  Vl0=-282.696
      settings: SourceProductBaseCode=PS
  Variable Resistor : spsVariableResistorLib/Variable Resistor  Rabsmin=20
      settings: SourceProductBaseCode=PS
  V+ : PMIOPort  Side=Right
  V- : PMIOPort  Port=2  Side=Right
  wires:
  R_signal/1 -> Variable Resistor/1
  L_signal/1 -> Variable Inductor/1
  connections:
  Variable Inductor/LConn1 -- V+/RConn1 -- Variable Resistor/LConn1
  V-/RConn1 -- Variable Resistor/RConn1 -- Variable Inductor/RConn1

== system LV_grid/RL_Load43 ==
  L_signal : Inport
  R_signal : Inport  Port=2
  Variable Inductor : spsVariableInductorLib/Variable Inductor  methode=Backward Euler  Labsmin=0.06  Initialize=off  iL0=0  L0=1e-3  Vl0=282.6909
      settings: SourceProductBaseCode=PS
  Variable Resistor : spsVariableResistorLib/Variable Resistor  Rabsmin=20
      settings: SourceProductBaseCode=PS
  V+ : PMIOPort  Side=Right
  V- : PMIOPort  Port=2  Side=Right
  wires:
  R_signal/1 -> Variable Resistor/1
  L_signal/1 -> Variable Inductor/1
  connections:
  Variable Inductor/LConn1 -- V+/RConn1 -- Variable Resistor/LConn1
  V-/RConn1 -- Variable Resistor/RConn1 -- Variable Inductor/RConn1

== system LV_grid/RL_Load44 ==
  L_signal : Inport
  R_signal : Inport  Port=2
  Variable Inductor : spsVariableInductorLib/Variable Inductor  methode=Backward Euler  Labsmin=0.06  Initialize=off  iL0=0  L0=1e-3  Vl0=282.8043
      settings: SourceProductBaseCode=PS
  Variable Resistor : spsVariableResistorLib/Variable Resistor  Rabsmin=20
      settings: SourceProductBaseCode=PS
  V+ : PMIOPort  Side=Right
  V- : PMIOPort  Port=2  Side=Right
  wires:
  R_signal/1 -> Variable Resistor/1
  L_signal/1 -> Variable Inductor/1
  connections:
  Variable Inductor/LConn1 -- V+/RConn1 -- Variable Resistor/LConn1
  V-/RConn1 -- Variable Resistor/RConn1 -- Variable Inductor/RConn1

== system LV_grid/RL_Load45 ==
  L_signal : Inport
  R_signal : Inport  Port=2
  Variable Inductor : spsVariableInductorLib/Variable Inductor  methode=Backward Euler  Labsmin=0.06  Initialize=off  iL0=0  L0=1e-3  Vl0=-282.6598
      settings: SourceProductBaseCode=PS
  Variable Resistor : spsVariableResistorLib/Variable Resistor  Rabsmin=20
      settings: SourceProductBaseCode=PS
  V+ : PMIOPort  Side=Right
  V- : PMIOPort  Port=2  Side=Right
  wires:
  R_signal/1 -> Variable Resistor/1
  L_signal/1 -> Variable Inductor/1
  connections:
  Variable Inductor/LConn1 -- V+/RConn1 -- Variable Resistor/LConn1
  V-/RConn1 -- Variable Resistor/RConn1 -- Variable Inductor/RConn1

== system LV_grid/RL_Load46 ==
  L_signal : Inport
  R_signal : Inport  Port=2
  Variable Inductor : spsVariableInductorLib/Variable Inductor  methode=Backward Euler  Labsmin=0.06  Initialize=off  iL0=0  L0=1e-3  Vl0=-0.055655
      settings: SourceProductBaseCode=PS
  Variable Resistor : spsVariableResistorLib/Variable Resistor  Rabsmin=20
      settings: SourceProductBaseCode=PS
  V+ : PMIOPort  Side=Right
  V- : PMIOPort  Port=2  Side=Right
  wires:
  R_signal/1 -> Variable Resistor/1
  L_signal/1 -> Variable Inductor/1
  connections:
  Variable Inductor/LConn1 -- V+/RConn1 -- Variable Resistor/LConn1
  V-/RConn1 -- Variable Resistor/RConn1 -- Variable Inductor/RConn1

== system LV_grid/RL_Load47 ==
  L_signal : Inport
  R_signal : Inport  Port=2
  Variable Inductor : spsVariableInductorLib/Variable Inductor  methode=Backward Euler  Labsmin=0.06  Initialize=off  iL0=0  L0=1e-3  Vl0=-0.054761
      settings: SourceProductBaseCode=PS
  Variable Resistor : spsVariableResistorLib/Variable Resistor  Rabsmin=20
      settings: SourceProductBaseCode=PS
  V+ : PMIOPort  Side=Right
  V- : PMIOPort  Port=2  Side=Right
  wires:
  R_signal/1 -> Variable Resistor/1
  L_signal/1 -> Variable Inductor/1
  connections:
  Variable Inductor/LConn1 -- V+/RConn1 -- Variable Resistor/LConn1
  V-/RConn1 -- Variable Resistor/RConn1 -- Variable Inductor/RConn1

== system LV_grid/RL_Load5 ==
  L_signal : Inport
  R_signal : Inport  Port=2
  Variable Inductor : spsVariableInductorLib/Variable Inductor  methode=Backward Euler  Labsmin=0.06  Initialize=off  iL0=0  L0=1e-3  Vl0=-0.05675
      settings: SourceProductBaseCode=PS
  Variable Resistor : spsVariableResistorLib/Variable Resistor  Rabsmin=20
      settings: SourceProductBaseCode=PS
  V+ : PMIOPort  Side=Right
  V- : PMIOPort  Port=2  Side=Right
  wires:
  R_signal/1 -> Variable Resistor/1
  L_signal/1 -> Variable Inductor/1
  connections:
  Variable Inductor/LConn1 -- V+/RConn1 -- Variable Resistor/LConn1
  V-/RConn1 -- Variable Resistor/RConn1 -- Variable Inductor/RConn1

== system LV_grid/RL_Load6 ==
  L_signal : Inport
  R_signal : Inport  Port=2
  Variable Inductor : spsVariableInductorLib/Variable Inductor  methode=Backward Euler  Labsmin=0.06  Initialize=off  iL0=0  L0=1e-3  Vl0=-282.7103
      settings: SourceProductBaseCode=PS
  Variable Resistor : spsVariableResistorLib/Variable Resistor  Rabsmin=20
      settings: SourceProductBaseCode=PS
  V+ : PMIOPort  Side=Right
  V- : PMIOPort  Port=2  Side=Right
  wires:
  R_signal/1 -> Variable Resistor/1
  L_signal/1 -> Variable Inductor/1
  connections:
  Variable Inductor/LConn1 -- V+/RConn1 -- Variable Resistor/LConn1
  V-/RConn1 -- Variable Resistor/RConn1 -- Variable Inductor/RConn1

== system LV_grid/RL_Load7 ==
  L_signal : Inport
  R_signal : Inport  Port=2
  Variable Inductor : spsVariableInductorLib/Variable Inductor  methode=Backward Euler  Labsmin=0.06  Initialize=off  iL0=0  L0=1e-3  Vl0=282.8029
      settings: SourceProductBaseCode=PS
  Variable Resistor : spsVariableResistorLib/Variable Resistor  Rabsmin=20
      settings: SourceProductBaseCode=PS
  V+ : PMIOPort  Side=Right
  V- : PMIOPort  Port=2  Side=Right
  wires:
  R_signal/1 -> Variable Resistor/1
  L_signal/1 -> Variable Inductor/1
  connections:
  Variable Inductor/LConn1 -- V+/RConn1 -- Variable Resistor/LConn1
  V-/RConn1 -- Variable Resistor/RConn1 -- Variable Inductor/RConn1

== system LV_grid/RL_Load8 ==
  L_signal : Inport
  R_signal : Inport  Port=2
  Variable Inductor : spsVariableInductorLib/Variable Inductor  methode=Backward Euler  Labsmin=0.06  Initialize=off  iL0=0  L0=1e-3  Vl0=-282.6182
      settings: SourceProductBaseCode=PS
  Variable Resistor : spsVariableResistorLib/Variable Resistor  Rabsmin=20
      settings: SourceProductBaseCode=PS
  V+ : PMIOPort  Side=Right
  V- : PMIOPort  Port=2  Side=Right
  wires:
  R_signal/1 -> Variable Resistor/1
  L_signal/1 -> Variable Inductor/1
  connections:
  Variable Inductor/LConn1 -- V+/RConn1 -- Variable Resistor/LConn1
  V-/RConn1 -- Variable Resistor/RConn1 -- Variable Inductor/RConn1

== system LV_grid/RL_Load9 ==
  L_signal : Inport
  R_signal : Inport  Port=2
  Variable Inductor : spsVariableInductorLib/Variable Inductor  methode=Backward Euler  Labsmin=0.06  Initialize=off  iL0=0  L0=1e-3  Vl0=282.8052
      settings: SourceProductBaseCode=PS
  Variable Resistor : spsVariableResistorLib/Variable Resistor  Rabsmin=20
      settings: SourceProductBaseCode=PS
  V+ : PMIOPort  Side=Right
  V- : PMIOPort  Port=2  Side=Right
  wires:
  R_signal/1 -> Variable Resistor/1
  L_signal/1 -> Variable Inductor/1
  connections:
  Variable Inductor/LConn1 -- V+/RConn1 -- Variable Resistor/LConn1
  V-/RConn1 -- Variable Resistor/RConn1 -- Variable Inductor/RConn1

== system LV_grid/L1/L1 ==
  Pi Section Line : spsPiSectionLineLib/Pi Section Line  LConnTagsString=__new0  RConnTagsString=__new0  Phases=1  PiSections=1  Length=0.0025  Frequency=50  Resistance=0.274  Inductance=0.073  Capacitance=12.74e-9  Measurements=None  Measurements2=None
      settings: SourceProductBaseCode=PS
  Three-Phase PI Section Line : spsThreePhasePISectionLineLib/Three-Phase PI Section Line  LConnTagsString=a|b|c  RConnTagsString=A|B|C  Length=0.0025  Frequency=50  Resistances=[ 0.274 0.959]  Inductances=[ 0.073 0.079]  Capacitances=[12.74e-9 7.751e-9]
  A : PMIOPort  Side=Left
  B : PMIOPort  Port=2  Side=Left
  C : PMIOPort  Port=3  Side=Left
  N : PMIOPort  Port=4  Side=Left
  a : PMIOPort  Port=5  Side=Right
  b : PMIOPort  Port=6  Side=Right
  c : PMIOPort  Port=7  Side=Right
  n : PMIOPort  Port=8  Side=Right
  connections:
  Pi Section Line/LConn1 -- N/RConn1
  Pi Section Line/RConn1 -- n/RConn1
  C/RConn1 -- Three-Phase PI Section Line/LConn3
  B/RConn1 -- Three-Phase PI Section Line/LConn2
  A/RConn1 -- Three-Phase PI Section Line/LConn1
  Three-Phase PI Section Line/RConn3 -- c/RConn1
  Three-Phase PI Section Line/RConn2 -- b/RConn1
  Three-Phase PI Section Line/RConn1 -- a/RConn1

== system LV_grid/L10/L1 ==
  Pi Section Line : spsPiSectionLineLib/Pi Section Line  LConnTagsString=__new0  RConnTagsString=__new0  Phases=1  PiSections=1  Length=0.0025  Frequency=50  Resistance=0.274  Inductance=0.073  Capacitance=12.74e-9  Measurements=None  Measurements2=None
      settings: SourceProductBaseCode=PS
  Three-Phase PI Section Line : spsThreePhasePISectionLineLib/Three-Phase PI Section Line  LConnTagsString=a|b|c  RConnTagsString=A|B|C  Length=0.0025  Frequency=50  Resistances=[ 0.274 0.959]  Inductances=[ 0.073 0.079]  Capacitances=[12.74e-9 7.751e-9]
  A : PMIOPort  Side=Left
  B : PMIOPort  Port=2  Side=Left
  C : PMIOPort  Port=3  Side=Left
  N : PMIOPort  Port=4  Side=Left
  a : PMIOPort  Port=5  Side=Right
  b : PMIOPort  Port=6  Side=Right
  c : PMIOPort  Port=7  Side=Right
  n : PMIOPort  Port=8  Side=Right
  connections:
  Pi Section Line/LConn1 -- N/RConn1
  Pi Section Line/RConn1 -- n/RConn1
  C/RConn1 -- Three-Phase PI Section Line/LConn3
  B/RConn1 -- Three-Phase PI Section Line/LConn2
  A/RConn1 -- Three-Phase PI Section Line/LConn1
  Three-Phase PI Section Line/RConn3 -- c/RConn1
  Three-Phase PI Section Line/RConn2 -- b/RConn1
  Three-Phase PI Section Line/RConn1 -- a/RConn1
